simulink model "RLS_2018a"  (R2020b)
settings: Solver=VariableStepAuto  StartTime=0.0  StopTime=6000  RelTol=1e-3  EnableMultiTasking=on
values from neighbouring files (symbols this model uses):
  A = [1 -1.6 0.64]    [init_RLS.m]
  alpha = 1    [init_RLS.m]
  B = [0 0 0.15]    [init_RLS.m]
  K = 200    [init_RLS.m]
  lambda = 0.995    [init_RLS.m]
  P_0 = eye(3,3)*1    [init_RLS.m]
  Theta_hat_0 = [0 0 0]'    [init_RLS.m]
settings Model: Creator=thomas.schauer  LastModifiedBy=schauer
settings DataIOCC: LimitDataPoints=on  ReturnWorkspaceOutputs=off
settings OptimizationCC: LifeSpan=inf
settings DebuggingCC: AllowSymbolicDim=off  SFUnexpectedBacktrackingDiag=warning  SFNoUnconditionalDefaultTransitionDiag=warning  SFExecutionAtInitializationDiag=none  ArithmeticOperatorsInVariantConditions=warning
settings ModelReferenceCC: PropagateSignalLabelsOutOfModel=off
settings SFSimCC: SimUseLocalCustomCode=off  CustomCodeUndefinedFunction=UseInterfaceOnly
settings RTWCC: RTWUseLocalCustomCode=off
settings CodeAppCC: StateflowObjectComments=on
settings GRTTargetCC: TargetLangStandard=C89/C90 (ANSI)
settings ConfigComp: CovMetricSettings=dw  CovSaveCumulativeToWorkspaceVar=on  CovSaveSingleToWorkspaceVar=on  CovExternalEMLEnable=off

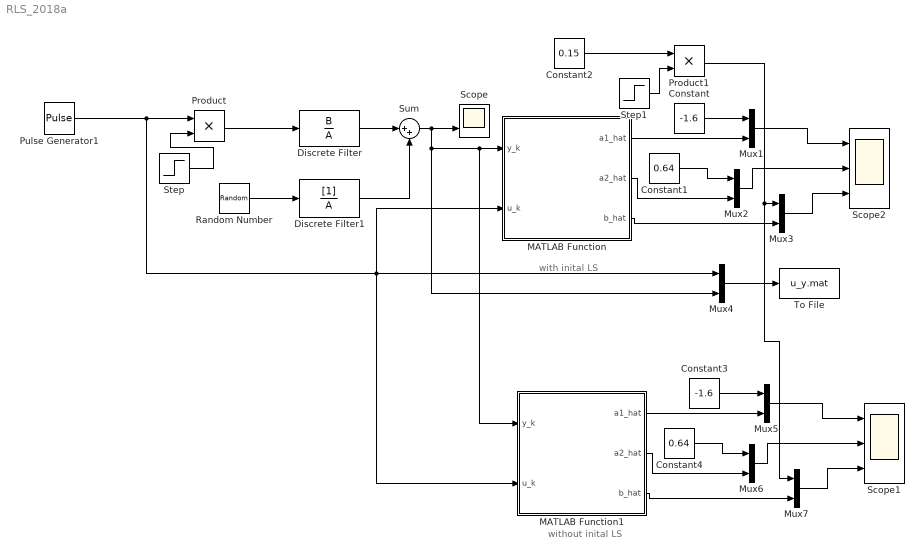
== system RLS_2018a ==
  note: with inital LS
  note: without inital LS
  Constant : Constant  Value=-1.6
  Constant1 : Constant  Value=0.64
  Constant2 : Constant  Value=0.15
  Constant3 : Constant  Value=-1.6
  Constant4 : Constant  Value=0.64
  Discrete Filter : DiscreteFilter  Numerator=B  Denominator=A  SampleTime=1
  Discrete Filter1 : DiscreteFilter  Denominator=A  SampleTime=1
  MATLAB Function : MATLAB Function  TreatAsAtomicUnit=on  SystemSampleTime=1
  MATLAB Function1 : MATLAB Function  TreatAsAtomicUnit=on  SystemSampleTime=1
  Mux{1..7} (7 alike) : Mux  Inputs=2
  Product : Product
  Product1 : Product
  Pulse Generator1 : DiscretePulseGenerator  PulseType=Time based  Period=100  PulseWidth=50
  Random Number : RandomNumber  Variance=0.1^2  SampleTime=1
  Scope : Scope  NumInputPorts=2
  Scope1 : Scope  NumInputPorts=3
  Scope2 : Scope  NumInputPorts=3
  Step : Step  Time=3000  Before=1  After=2  SampleTime=0
  Step1 : Step  Time=3000  Before=1  After=2  SampleTime=0
  Sum : Sum  Inputs=|++
  To File : ToFile  Filename=u_y.mat  SaveFormat=Timeseries
  wires:
  Pulse Generator1/1 -> Product/1, MATLAB Function1/2(u_k), MATLAB Function/2(u_k), Mux4/1
  Discrete Filter/1 -> Sum/1
  Discrete Filter1/1 -> Sum/2
  Random Number/1 -> Discrete Filter1/1
  Sum/1 -> Mux4/2, MATLAB Function1/1(y_k), MATLAB Function/1(y_k), Scope/2
  MATLAB Function/1(a1_hat) -> Mux1/2
  MATLAB Function/2(a2_hat) -> Mux2/2
  MATLAB Function/3(b_hat) -> Mux3/2
  Mux3/1 -> Scope2/3
  Mux2/1 -> Scope2/2
  Mux1/1 -> Scope2/1
  Constant1/1 -> Mux2/1
  Constant/1 -> Mux1/1
  Mux4/1 -> To File/1
  MATLAB Function1/1(a1_hat) -> Mux5/2
  Mux6/1 -> Scope1/2
  MATLAB Function1/2(a2_hat) -> Mux6/2
  Mux5/1 -> Scope1/1
  Constant3/1 -> Mux5/1
  Mux7/1 -> Scope1/3
  Constant4/1 -> Mux6/1
  MATLAB Function1/3(b_hat) -> Mux7/2
  Product1/1 -> Mux7/1, Mux3/1
  Step/1 -> Product/2
  Product/1 -> Discrete Filter/1
  Constant2/1 -> Product1/1
  Step1/1 -> Product1/2

== matlab function RLS_2018a/MATLAB Function1 ==
  data: y_k input; a1_hat output; u_k input; Theta_hat_0 parameter; P_0 parameter; lambda parameter; a2_hat output; b_hat output; alpha parameter
function [a1_hat,a2_hat,b_hat] = fcn(y_k,u_k,Theta_hat_0,P_0,lambda, alpha)
persistent  Theta_hat_km1 u_km1 u_km2 y_km1 y_km2 P_km1

%Initialisation
if isempty(Theta_hat_km1) 
    %for RLS
    P_km1=P_0;
    Theta_hat_km1=Theta_hat_0;
    u_km1=0;u_km2=0;y_km1=0;y_km2=0;
end

phi_k=[-y_km1 -y_km2 u_km2]';
L=(P_km1*phi_k)/(lambda/alpha+phi_k'*P_km1*phi_k);
    
Theta_hat_k = Theta_hat_km1 + L*(y_k-phi_k'*Theta_hat_km1);
P_k=1/lambda*(P_km1-L*phi_k'*P_km1);

a1_hat=Theta_hat_k(1);
a2_hat=Theta_hat_k(2);
b_hat=Theta_hat_k(3);

P_km1=P_k;
y_km2=y_km1;y_km1=y_k;
u_km2=u_km1;u_km1=u_k;
Theta_hat_km1=Theta_hat_k;

== matlab function RLS_2018a/MATLAB Function ==
  data: y_k input; a1_hat output; u_k input; Theta_hat_0 parameter; P_0 parameter; lambda parameter; a2_hat output; b_hat output; K parameter; alpha parameter
function [a1_hat,a2_hat,b_hat] = fcn(y_k,u_k,Theta_hat_0,P_0,lambda,K,alpha)
persistent  Theta_hat_km1 u_km1 u_km2 y_km1 y_km2 P_km1 i PHI Y;

%Initialisation
if isempty(Theta_hat_km1) 
    %for RLS
    Theta_hat_km1=Theta_hat_0;
    P_km1=P_0;
    u_km1=0;u_km2=0;y_km1=0;y_km2=0;
    %for initial LS
    PHI=zeros(K,length(Theta_hat_0));
    Y=zeros(K,1);
    i=1;
end


phi_k=[-y_km1 -y_km2 u_km2]';
L=(P_km1*phi_k)/(lambda/alpha+phi_k'*P_km1*phi_k);
    
if i>K %normal RLS after LS has finished and determined the P0,Theta_hat_0    
    Theta_hat_k = Theta_hat_km1 + L*(y_k-phi_k'*Theta_hat_km1);
    P_k=1/lambda*(P_km1-L*phi_k'*P_km1);
elseif i==K %collect final data and perform LS
    PHI(i,:)=phi_k';
    Y(i,:)=y_k;    
    Theta_hat_k=PHI\Y;
    P_k=inv(PHI'*PHI);
else %collect data
    PHI(i,:)=phi_k';
    Y(i,:)=y_k;
    Theta_hat_k=Theta_hat_0;
    P_k=P_0;
end

a1_hat=Theta_hat_k(1);
a2_hat=Theta_hat_k(2);
b_hat=Theta_hat_k(3);

P_km1=P_k;
y_km2=y_km1;y_km1=y_k;
u_km2=u_km1;u_km1=u_k;
Theta_hat_km1=Theta_hat_k;
i=i+1;
